simulink model "untitled"  (R2016b)
settings: Solver=ode4  StartTime=0.0  StopTime=1  FixedStep=0.01  RelTol=1e-3
libraries: simulink x1
settings Model: Creator=a029799  LastModifiedBy=a029799

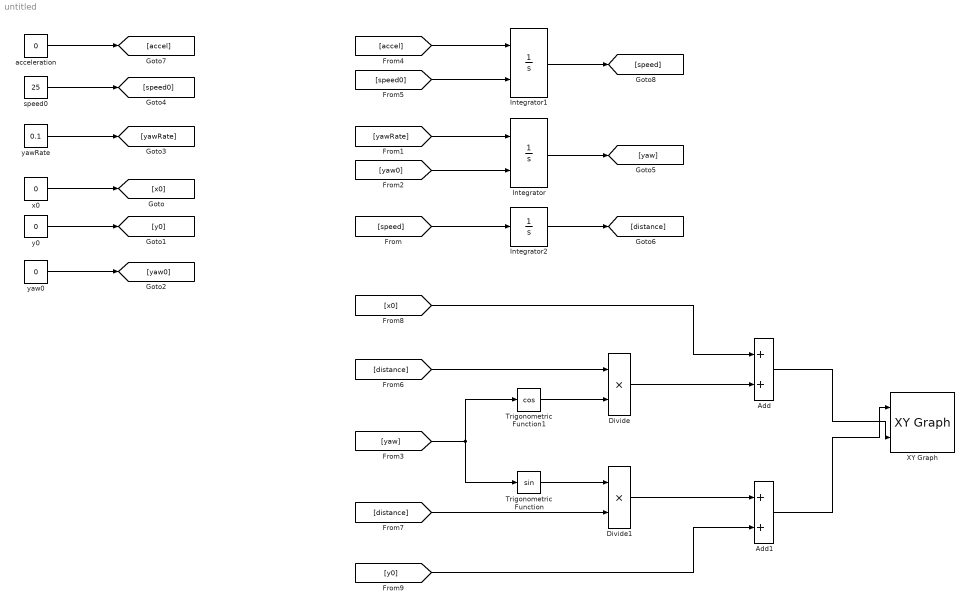
== system untitled ==
  Add : Sum
  Add1 : Sum
  Divide : Product  Inputs=**
  Divide1 : Product  Inputs=**
  Integrator : Integrator  InitialConditionSource=external
  Integrator1 : Integrator  InitialConditionSource=external
  Integrator2 : Integrator
  Trigonometric Function : Trigonometry
  Trigonometric Function1 : Trigonometry  Operator=cos
  XY Graph : simulink/Sinks/XY Graph  xmin=-1000  xmax=1000  ymin=-1000  ymax=1000  st=-1
  acceleration : Constant  Value=0
  speed0 : Constant  Value=25
  x0 : Constant  Value=0
  y0 : Constant  Value=0
  yaw0 : Constant  Value=0
  yawRate : Constant  Value=0.1
  wires:
  x0/1 -> [x0]
  y0/1 -> [y0]
  yaw0/1 -> [yaw0]
  yawRate/1 -> [yawRate]
  speed0/1 -> [speed0]
  [yaw0] -> Integrator/2
  [yawRate] -> Integrator/1
  Integrator/1 -> [yaw]
  [yaw] -> Trigonometric Function1/1, Trigonometric Function/1
  Trigonometric Function1/1 -> Divide/2
  Trigonometric Function/1 -> Divide1/1
  [speed0] -> Integrator1/2
  [accel] -> Integrator1/1
  Integrator1/1 -> [speed]
  acceleration/1 -> [accel]
  [speed] -> Integrator2/1
  Integrator2/1 -> [distance]
  [distance] -> Divide/1
  [distance] -> Divide1/2
  Divide/1 -> Add/2
  [x0] -> Add/1
  Divide1/1 -> Add1/1
  [y0] -> Add1/2
  Add/1 -> XY Graph/2
  Add1/1 -> XY Graph/1
